simulink model "garage_parking"  (R2019b)
settings: Solver=VariableStepAuto  StartTime=0.0  StopTime=20.0  RelTol=1e-3
undefined symbols (not defined in the file): delta_max, parking_speed, TOF_distance_limit
libraries: simulink x4

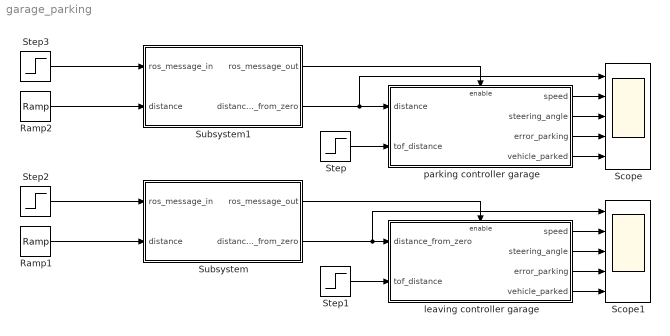
== system garage_parking ==
  Ramp1 : simulink/Sources/Ramp  slope=100  start=0  InitialOutput=0
  Ramp2 : simulink/Sources/Ramp  slope=100  start=0  InitialOutput=0
  Scope : Scope  NumInputPorts=5
  Scope1 : Scope  NumInputPorts=5
  Step : Step  Time=12  Before=30  SampleTime=0
  Step1 : Step  Time=12  Before=30  SampleTime=0
  Step2 : Step  Time=3  SampleTime=0
  Step3 : Step  Time=3  SampleTime=0
  Subsystem : Subsystem
  Subsystem1 : Subsystem
  leaving controller garage : Subsystem
  parking controller garage : Subsystem
  wires:
  parking controller garage/1(speed) -> Scope/2
  parking controller garage/2(steering_angle) -> Scope/3
  parking controller garage/3(error_parking) -> Scope/4
  parking controller garage/4("vehicle_parked ") -> Scope/5
  leaving controller garage/1(speed) -> Scope1/2
  leaving controller garage/2(steering_angle) -> Scope1/3
  leaving controller garage/3(error_parking) -> Scope1/4
  leaving controller garage/4("vehicle_parked ") -> Scope1/5
  Step2/1 -> Subsystem/1(ros_message_in)
  Step1/1 -> leaving controller garage/2(tof_distance)
  Step/1 -> parking controller garage/2(tof_distance)
  Subsystem/2(distance_from_zero) -> Scope1/1, leaving controller garage/1(distance_from_zero)
  Ramp1/1 -> Subsystem/2(distance)
  Subsystem/1("ros_message_out ") -> leaving controller garage/Enable
  Step3/1 -> Subsystem1/1(ros_message_in)
  Ramp2/1 -> Subsystem1/2(distance)
  Subsystem1/2(distance_from_zero) -> Scope/1, parking controller garage/1(distance)
  Subsystem1/1("ros_message_out ") -> parking controller garage/Enable

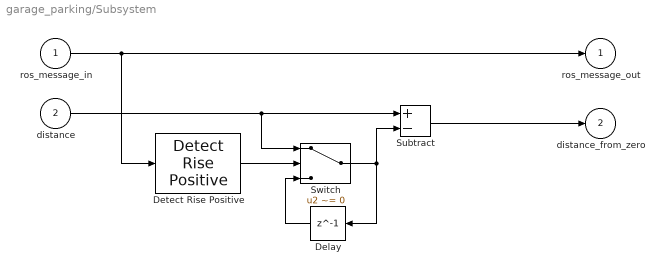
== system garage_parking/Subsystem ==
  ros_message_in : Inport
  distance : Inport  Port=2
  Delay : Delay  DelayLength=1
  "Detect Rise Positive " : simulink/Logic and Bit Operations/Detect Rise Positive  vinit=0  OutDataTypeStr=boolean
  Subtract : Sum  Inputs=+-
  Switch : Switch  Criteria=u2 ~= 0
  "ros_message_out " : Outport
  distance_from_zero : Outport  Port=2
  wires:
  ros_message_in/1 -> "Detect Rise Positive "/1, "ros_message_out "/1
  Delay/1 -> Switch/3
  Subtract/1 -> distance_from_zero/1
  distance/1 -> Switch/1, Subtract/1
  Switch/1 -> Subtract/2, Delay/1
  "Detect Rise Positive "/1 -> Switch/2

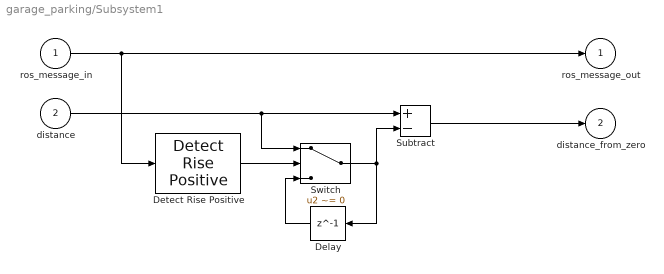
== system garage_parking/Subsystem1 ==
  ros_message_in : Inport
  distance : Inport  Port=2
  Delay : Delay  DelayLength=1
  "Detect Rise Positive " : simulink/Logic and Bit Operations/Detect Rise Positive  vinit=0  OutDataTypeStr=boolean
  Subtract : Sum  Inputs=+-
  Switch : Switch  Criteria=u2 ~= 0
  "ros_message_out " : Outport
  distance_from_zero : Outport  Port=2
  wires:
  ros_message_in/1 -> "Detect Rise Positive "/1, "ros_message_out "/1
  Delay/1 -> Switch/3
  Subtract/1 -> distance_from_zero/1
  distance/1 -> Switch/1, Subtract/1
  Switch/1 -> Subtract/2, Delay/1
  "Detect Rise Positive "/1 -> Switch/2

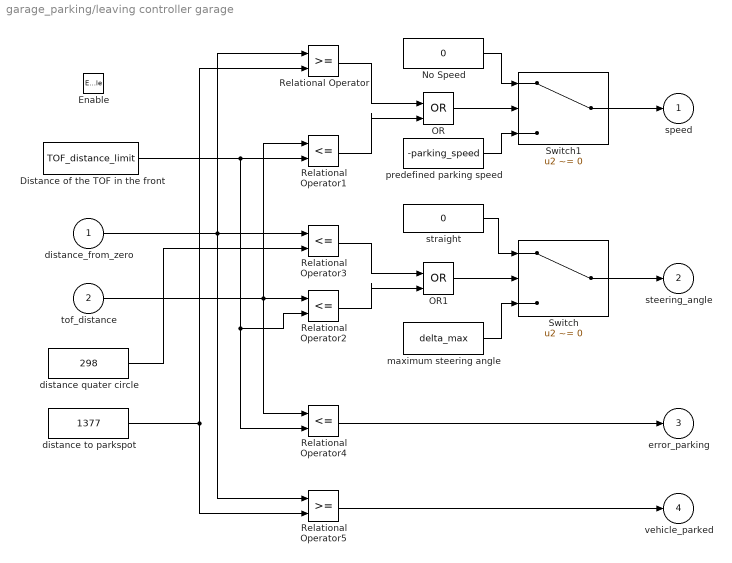
== system garage_parking/leaving controller garage ==
  distance_from_zero : Inport
  tof_distance : Inport  Port=2
  Enable : EnablePort
  "Distance of the TOF in the front " : Constant  Value=TOF_distance_limit
  No Speed : Constant  Value=0
  OR : Logic  Operator=OR  IconShape=distinctive  AllPortsSameDT=off  OutDataTypeStr=boolean
  OR1 : Logic  Operator=OR  IconShape=distinctive  AllPortsSameDT=off  OutDataTypeStr=boolean
  Relational Operator : RelationalOperator  OutDataTypeStr=boolean  RndMeth=Simplest
  Relational Operator{1..4} (4 alike) : RelationalOperator  Operator=<=  OutDataTypeStr=boolean  RndMeth=Simplest
  Relational Operator5 : RelationalOperator  OutDataTypeStr=boolean  RndMeth=Simplest
  Switch : Switch  Criteria=u2 ~= 0  Threshold=1079  OutDataTypeStr=single
  Switch1 : Switch  Criteria=u2 ~= 0  Threshold=1377  OutDataTypeStr=single
  "distance quater circle " : Constant  Value=298
  distance to parkspot : Constant  Value=1377
  maximum steering angle : Constant  Value=delta_max
  predefined parking speed : Constant  Value=-parking_speed
  straight : Constant  Value=0
  speed : Outport
  steering_angle : Outport  Port=2
  error_parking : Outport  Port=3
  "vehicle_parked " : Outport  Port=4
  wires:
  Switch1/1 -> speed/1
  Switch/1 -> steering_angle/1
  straight/1 -> Switch/1
  maximum steering angle/1 -> Switch/3
  No Speed/1 -> Switch1/1
  predefined parking speed/1 -> Switch1/3
  Relational Operator/1 -> OR/1
  OR/1 -> Switch1/2
  Relational Operator1/1 -> OR/2
  tof_distance/1 -> Relational Operator4/1, Relational Operator2/1, Relational Operator1/1
  Relational Operator2/1 -> OR1/2
  "distance quater circle "/1 -> Relational Operator3/2
  Relational Operator3/1 -> OR1/1
  OR1/1 -> Switch/2
  "Distance of the TOF in the front "/1 -> Relational Operator4/2, Relational Operator2/2, Relational Operator1/2
  Relational Operator4/1 -> error_parking/1
  distance_from_zero/1 -> Relational Operator/1, Relational Operator5/1, Relational Operator3/1
  distance to parkspot/1 -> Relational Operator5/2, Relational Operator/2
  Relational Operator5/1 -> "vehicle_parked "/1

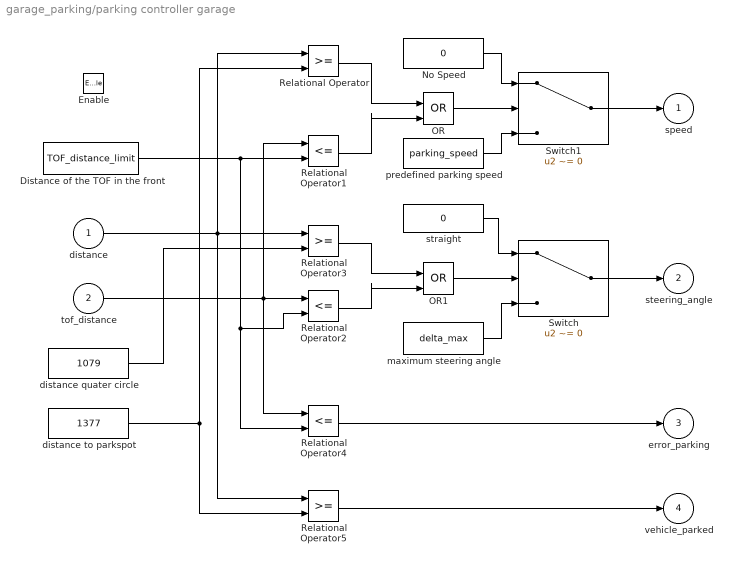
== system garage_parking/parking controller garage ==
  distance : Inport
  tof_distance : Inport  Port=2
  Enable : EnablePort
  "Distance of the TOF in the front " : Constant  Value=TOF_distance_limit
  No Speed : Constant  Value=0
  OR : Logic  Operator=OR  IconShape=distinctive  AllPortsSameDT=off  OutDataTypeStr=boolean
  OR1 : Logic  Operator=OR  IconShape=distinctive  AllPortsSameDT=off  OutDataTypeStr=boolean
  Relational Operator : RelationalOperator  OutDataTypeStr=boolean  RndMeth=Simplest
  Relational Operator1 : RelationalOperator  Operator=<=  OutDataTypeStr=boolean  RndMeth=Simplest
  Relational Operator2 : RelationalOperator  Operator=<=  OutDataTypeStr=boolean  RndMeth=Simplest
  Relational Operator3 : RelationalOperator  OutDataTypeStr=boolean  RndMeth=Simplest
  Relational Operator4 : RelationalOperator  Operator=<=  OutDataTypeStr=boolean  RndMeth=Simplest
  Relational Operator5 : RelationalOperator  OutDataTypeStr=boolean  RndMeth=Simplest
  Switch : Switch  Criteria=u2 ~= 0  Threshold=1079  OutDataTypeStr=single
  Switch1 : Switch  Criteria=u2 ~= 0  Threshold=1377  OutDataTypeStr=single
  "distance quater circle " : Constant  Value=1079
  distance to parkspot : Constant  Value=1377
  maximum steering angle : Constant  Value=delta_max
  predefined parking speed : Constant  Value=parking_speed
  straight : Constant  Value=0
  speed : Outport
  steering_angle : Outport  Port=2
  error_parking : Outport  Port=3
  "vehicle_parked " : Outport  Port=4
  wires:
  Switch1/1 -> speed/1
  Switch/1 -> steering_angle/1
  straight/1 -> Switch/1
  maximum steering angle/1 -> Switch/3
  No Speed/1 -> Switch1/1
  predefined parking speed/1 -> Switch1/3
  Relational Operator/1 -> OR/1
  OR/1 -> Switch1/2
  Relational Operator1/1 -> OR/2
  tof_distance/1 -> Relational Operator4/1, Relational Operator2/1, Relational Operator1/1
  Relational Operator2/1 -> OR1/2
  "distance quater circle "/1 -> Relational Operator3/2
  Relational Operator3/1 -> OR1/1
  OR1/1 -> Switch/2
  "Distance of the TOF in the front "/1 -> Relational Operator4/2, Relational Operator2/2, Relational Operator1/2
  Relational Operator4/1 -> error_parking/1
  distance/1 -> Relational Operator/1, Relational Operator5/1, Relational Operator3/1
  distance to parkspot/1 -> Relational Operator5/2, Relational Operator/2
  Relational Operator5/1 -> "vehicle_parked "/1
